simulink model "Project1Week2_"  (R2023b)
settings: Solver=ode1  StartTime=0.0  StopTime=25  FixedStep=0.1  RelTol=1e-3
values from neighbouring files (symbols this model uses):
  A = 1    [Project1Week2.m]    (also in ProjectWeek1.m; Project_1.m = 4)
  b = 1    [Project1Week2.m]    (also in ProjectWeek1.m; Project_1.m)
  J = 1    [Project1Week2.m]    (also in ProjectWeek1.m; Project_1.m)
  w_0 = 1    [Project1Week2.m]    (also in ProjectWeek1.m; Project_1.m)
settings Model: Creator=Julian Tan  LastModifiedBy=Julian Tan

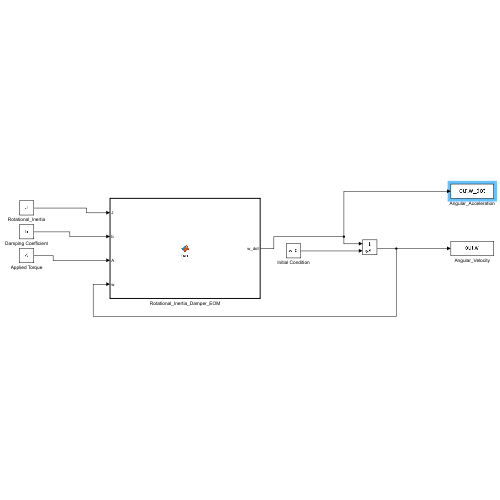
[thumbnail: Simulink's stored preview of the top-level diagram]
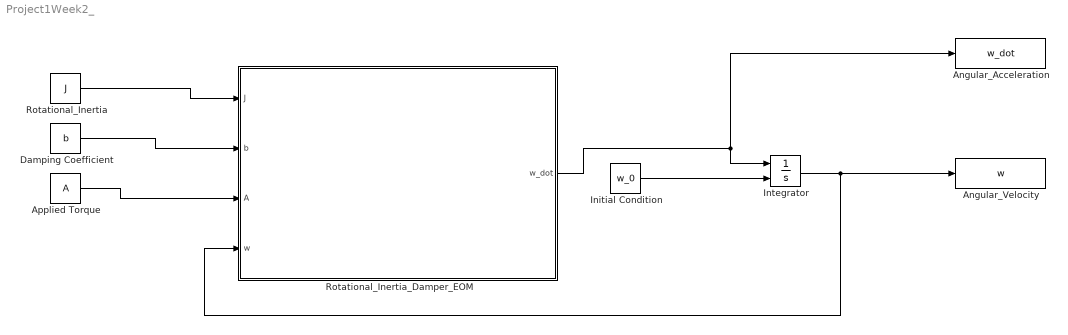
== system Project1Week2_ ==
  Angular_Acceleration : ToWorkspace  VariableName=w_dot  SaveFormat=Timeseries  SampleTime=-1
  Angular_Velocity : ToWorkspace  VariableName=w  SaveFormat=Timeseries  SampleTime=-1
  Applied Torque : Constant  Value=A
  Damping Coefficient : Constant  Value=b
  Initial Condition : Constant  Value=w_0
  Integrator : Integrator  InitialConditionSource=external
  Rotational_Inertia : Constant  Value=J
  Rotational_Inertia_Damper_EOM : MATLAB Function  TreatAsAtomicUnit=on
  wires:
  Rotational_Inertia_Damper_EOM/1(w_dot) -> Angular_Acceleration/1, Integrator/1
  Applied Torque/1 -> Rotational_Inertia_Damper_EOM/3(A)
  Initial Condition/1 -> Integrator/2
  Damping Coefficient/1 -> Rotational_Inertia_Damper_EOM/2(b)
  Integrator/1 -> Angular_Velocity/1, Rotational_Inertia_Damper_EOM/4(w)
  Rotational_Inertia/1 -> Rotational_Inertia_Damper_EOM/1(J)

== matlab function Project1Week2_/Rotational_Inertia_Damper_EOM ==
  data: J input; w_dot output; b input; A input; w input
function w_dot = fcn(J, b, A, w)

w_dot = (1/J)*(A-b*w);


end
